simulink model "SWEM_1"  (Simulink 8.6)
settings: Solver=FixedStepAuto  StartTime=0.0  StopTime=100  FixedStep=0.5  MaxStep=dt  RelTol=1e-3
undefined symbols (not defined in the file): fg, kx, ky, Om, phase, phig, PSI_swell, Ua
settings Model: Creator=brynljones  LastModifiedBy=brynljones
settings DataIOCC: SaveFormat=Dataset  SignalLoggingSaveFormat=Dataset
settings OptimizationCC: ExpressionDepthLimit=128
settings DebuggingCC: UnderspecifiedInitializationDetection=Simplified  MergeDetectMultiDrivingBlocksExec=error  SolverPrmCheckMsg=none  FcnCallInpInsideContextMsg=EnableAllAsError  StateNameClashWarn=none
settings HardwareCC: ProdBitPerPointer=64  ProdLargestAtomicFloat=Float  ProdIntDivRoundTo=Zero  ProdEndianess=LittleEndian  ProdWordSize=64  ProdHWDeviceType=Intel->x86-64 (Windows64)
settings GRTTargetCC: GeneratePreprocessorConditionals=Use local settings  CombineOutputUpdateFcns=on  GRTInterface=off
settings ConfigComp: CovModelRefEnable=off

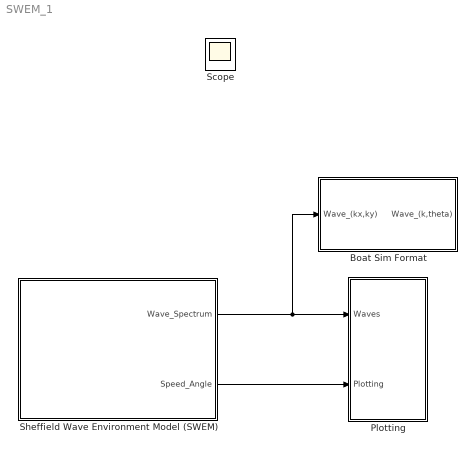
== system SWEM_1 ==
  Boat Sim Format : Subsystem
  Plotting : Subsystem
  Sheffield Wave Environment Model (SWEM) : Subsystem  mask{dt=0.5, M=256, Lx=100*pi, depth=1, lam=5, Viz=Surface Plot, Swell_Hs_u=Swell h_s, Hs_swell=1, U_swell=5, swell_angle=0, fetch_swell=1e10, U_mean=10, wind_angle=30, s=50, GF=1, df=1e-3, Nf=100, mu_wind=1, U_current=0.5, current_angle=-130, mu_current=1}
      mask prompts: dt "Time step (s):"; M "No. gridpoints:"; Lx "Dimension length (m):"; depth "Depth (m):"; lam "Choppy wave factor:"; Viz "Visualisation:"; Swell_Hs_u "Swell windspeed/fetch or h_s:"; Hs_swell "Swell h_s (m):"; U_swell "Swell windspeed (m/s):"; swell_angle "Swell angle (deg):"; fetch_swell "Swell fetch (m):"; U_mean "Mean local windspeed (m/s):"; wind_angle "Mean local wind angle (deg):"; s "Wind wave spreading (s):"; GF "Gust Factor:"; df "Gust freq. spacing:"; Nf "No. of gusting freq. components:"; mu_wind "Wind angle fluctuation coeff:"; U_current "Current speed (m/s):"; current_angle "Mean current angle (deg):"; mu_current "Current angle fluctuation coeff:"
      mask init:
      | if (Swell_Hs_u == 2)
      |     [Om,PSI_swell,kx,ky,phase,U_swell] = swellComponent_Hs(depth,M,M,Lx,Lx,Hs_swell,swell_angle);
      | else
      |     [Om,PSI_swell,kx,ky,phase] = swellComponent_U(depth,M,M,Lx,Lx,U_swell,fetch_swell,swell_angle);
      | end
      | [Ua,phig,fg] = Norso_Gust(U_mean,df,Nf);
      mask TypeOptions Viz: Surface Plot | Contour Plot | No Visualisation
      mask TypeOptions Swell_Hs_u: Swell windspeed/fetch | Swell h_s
      mask Display: image('sea1.jpg')
  Scope : Scope
  wires:
  Sheffield Wave Environment Model (SWEM)/1(Wave_Spectrum) -> Boat Sim Format/1(Wave_(kx,ky)), Plotting/1(Waves)
  Sheffield Wave Environment Model (SWEM)/2(Speed_Angle) -> Plotting/2(Plotting)

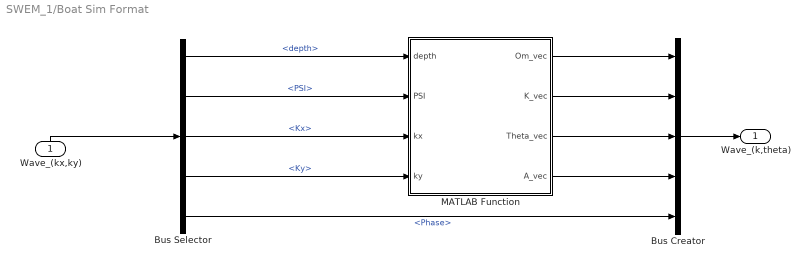
== system SWEM_1/Boat Sim Format ==
  Wave_(kx,ky) : Inport
  Bus Creator : BusCreator  Inputs=5
  Bus Selector : BusSelector  OutputSignals=depth,PSI,Kx,Ky,Phase
  MATLAB Function : MATLAB Function  TreatAsAtomicUnit=on
  Wave_(k,theta) : Outport
  wires:
  Bus Creator/1 -> Wave_(k,theta)/1
  MATLAB Function/2(K_vec) -> Bus Creator/2
  Bus Selector/3 -> MATLAB Function/3(kx)  "<Kx>"
  Bus Selector/4 -> MATLAB Function/4(ky)  "<Ky>"
  Wave_(kx,ky)/1 -> Bus Selector/1
  Bus Selector/2 -> MATLAB Function/2(PSI)  "<PSI>"
  Bus Selector/5 -> Bus Creator/5  "<Phase>"
  MATLAB Function/4(A_vec) -> Bus Creator/4
  MATLAB Function/3(Theta_vec) -> Bus Creator/3
  MATLAB Function/1(Om_vec) -> Bus Creator/1
  Bus Selector/1 -> MATLAB Function/1(depth)  "<depth>"

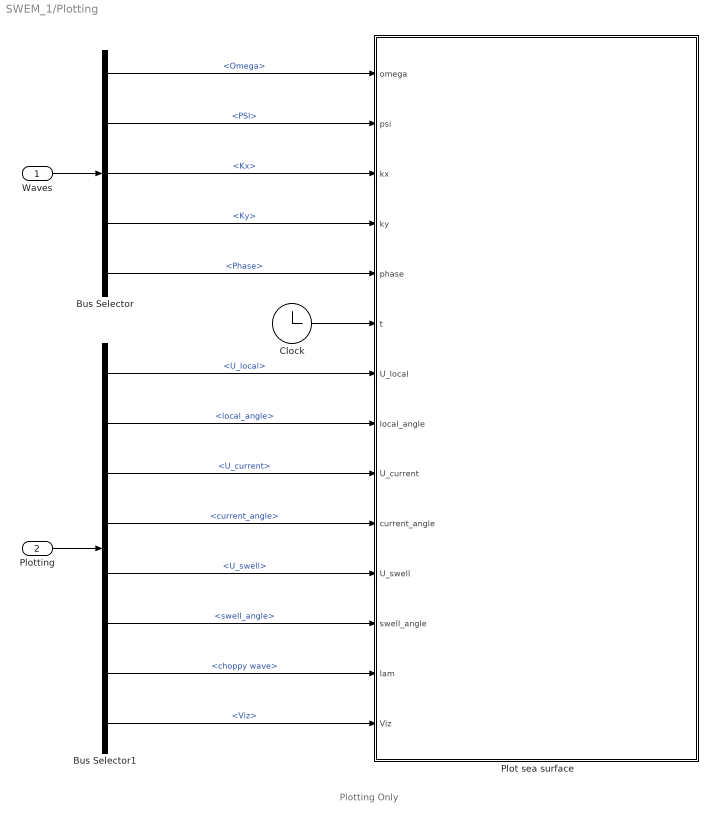
== system SWEM_1/Plotting ==
  note: Plotting Only
  Waves : Inport
  Plotting : Inport  Port=2
  Bus Selector : BusSelector  OutputSignals=Omega,PSI,Kx,Ky,Phase
  Bus Selector1 : BusSelector  OutputSignals=U_local,local_angle,U_current,current_angle,U_swell,swell_angle,choppy wave,Viz
  Clock : Clock
  Plot sea surface : MATLAB Function  TreatAsAtomicUnit=on
  wires:
  Waves/1 -> Bus Selector/1
  Bus Selector1/8 -> Plot sea surface/14(Viz)  "<Viz>"
  Bus Selector/3 -> Plot sea surface/3(kx)  "<Kx>"
  Bus Selector/4 -> Plot sea surface/4(ky)  "<Ky>"
  Bus Selector/5 -> Plot sea surface/5(phase)  "<Phase>"
  Bus Selector/2 -> Plot sea surface/2(psi)  "<PSI>"
  Bus Selector/1 -> Plot sea surface/1(omega)  "<Omega>"
  Plotting/1 -> Bus Selector1/1
  Clock/1 -> Plot sea surface/6(t)
  Bus Selector1/2 -> Plot sea surface/8(local_angle)  "<local_angle>"
  Bus Selector1/1 -> Plot sea surface/7(U_local)  "<U_local>"
  Bus Selector1/4 -> Plot sea surface/10(current_angle)  "<current_angle>"
  Bus Selector1/3 -> Plot sea surface/9(U_current)  "<U_current>"
  Bus Selector1/6 -> Plot sea surface/12(swell_angle)  "<swell_angle>"
  Bus Selector1/5 -> Plot sea surface/11(U_swell)  "<U_swell>"
  Bus Selector1/7 -> Plot sea surface/13(lam)  "<choppy wave>"

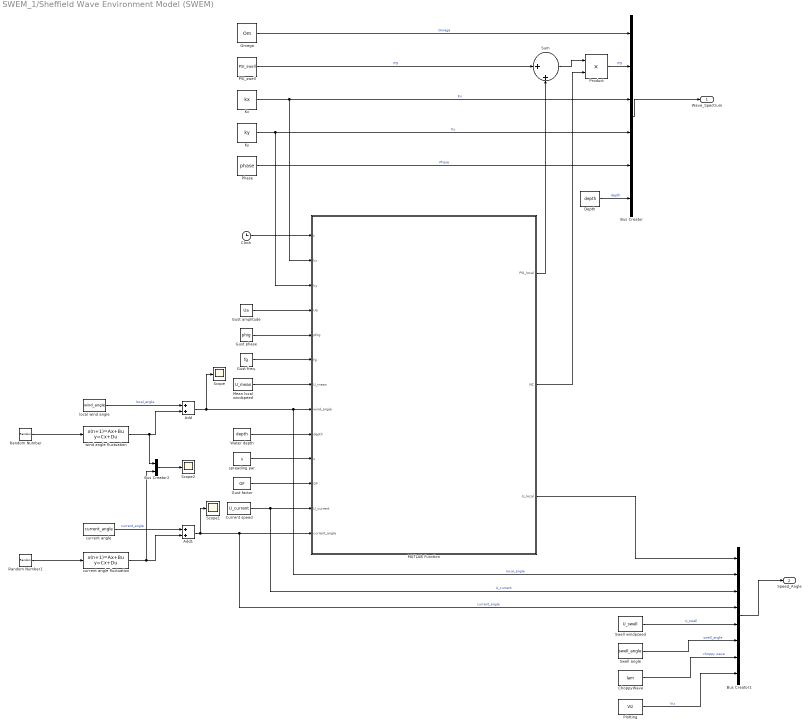
== system SWEM_1/Sheffield Wave Environment Model (SWEM) ==
  Add : Sum
  Add1 : Sum
  Bus Creator : BusCreator  Inputs=6
  Bus Creator1 : BusCreator  Inputs=8
  Bus Creator2 : BusCreator  Inputs=2
  ChoppyWave : Constant  Value=lam
  Clock : Clock
  Current speed : Constant  Value=U_current
  Depth : Constant  Value=depth
  Gust amplitude : Constant  Value=Ua
  Gust factor : Constant  Value=GF
  Gust freq. : Constant  Value=fg
  Gust phase : Constant  Value=phig
  Kx : Constant  Value=kx
  Ky : Constant  Value=ky
  MATLAB Function : MATLAB Function  TreatAsAtomicUnit=on
  Mean local windspeed : Constant  Value=U_mean
  Omega : Constant  Value=Om
  PSI_swell : Constant  Value=PSI_swell
  Phase : Constant  Value=phase
  Plotting : Constant  Value=Viz
  Product : Product
  Random Number : RandomNumber  Variance=5  Seed=2  SampleTime=dt
  Random Number1 : RandomNumber  Variance=2  Seed=1  SampleTime=dt
  Scope : Scope
  Scope1 : Scope
  Scope2 : Scope
  Sum : Sum  Inputs=|++
  Swell angle : Constant  Value=swell_angle
  Swell windpseed : Constant  Value=U_swell
  Water depth : Constant  Value=depth
  current angle : Constant  Value=current_angle
  current angle fluctuation : DiscreteStateSpace  A=1-(dt*mu_current)  B=dt  D=0  X0=-0.3  SampleTime=-1
  local wind angle : Constant  Value=wind_angle
  spreading par. : Constant  Value=s
  wind angle fluctuation : DiscreteStateSpace  A=1-(dt*mu_wind)  B=dt  D=0  X0=0.1  SampleTime=-1
  Wave_Spectrum : Outport
  Speed_Angle : Outport  Port=2
  wires:
  Ky/1 -> MATLAB Function/3(ky), Bus Creator/4  "Ky"
  Phase/1 -> Bus Creator/5  "Phase"
  Omega/1 -> Bus Creator/1  "Omega"
  Kx/1 -> MATLAB Function/2(kx), Bus Creator/3  "Kx"
  Bus Creator/1 -> Wave_Spectrum/1
  Clock/1 -> MATLAB Function/1(t)
  Gust amplitude/1 -> MATLAB Function/4(Ua)
  Gust phase/1 -> MATLAB Function/5(phig)
  Gust freq./1 -> MATLAB Function/6(fg)
  Mean local windspeed/1 -> MATLAB Function/7(U_mean)
  Water depth/1 -> MATLAB Function/9(depth)
  spreading par./1 -> MATLAB Function/10(s)
  Gust factor/1 -> MATLAB Function/11(GF)
  Current speed/1 -> Bus Creator1/3, MATLAB Function/12(U_current)  "U_current"
  MATLAB Function/1(PSI_local) -> Sum/2
  PSI_swell/1 -> Sum/1  "PSI"
  Product/1 -> Bus Creator/2  "PSI"
  MATLAB Function/2(NC) -> Product/2
  Sum/1 -> Product/1
  MATLAB Function/3(U_local) -> Bus Creator1/1
  Swell windpseed/1 -> Bus Creator1/5  "U_swell"
  Swell angle/1 -> Bus Creator1/6  "swell_angle"
  Bus Creator1/1 -> Speed_Angle/1
  Add/1 -> Scope/1, Bus Creator1/2, MATLAB Function/8(wind_angle)  "local_angle"
  local wind angle/1 -> Add/1  "local_angle"
  Random Number/1 -> wind angle fluctuation/1
  wind angle fluctuation/1 -> Bus Creator2/1, Add/2
  Random Number1/1 -> current angle fluctuation/1
  current angle/1 -> Add1/1  "current_angle"
  current angle fluctuation/1 -> Bus Creator2/2, Add1/2
  Add1/1 -> Scope1/1, Bus Creator1/4, MATLAB Function/13(current_angle)  "current_angle"
  Bus Creator2/1 -> Scope2/1
  ChoppyWave/1 -> Bus Creator1/7  "choppy wave"
  Plotting/1 -> Bus Creator1/8  "Viz"
  Depth/1 -> Bus Creator/6  "depth"

== matlab function Sheffield Wave Environment Model (SWEM)/MATLAB Function ==
  data: t input double; PSI_local output double; kx input double; ky input double; Ua input double; phig input double; fg input double; U_mean input double; wind_angle input double; depth input double; s input double; GF input double; U_current input double; current_angle input double; NC output double; U_local output double
function [PSI_local,NC,U_local] = fcn(t,kx,ky,Ua,phig,fg,U_mean,wind_angle,depth,s,GF,U_current,current_angle)
%#codegen


% calculate local wind = mean wind + gust
U_gust = sum(Ua.*cos(2*pi*fg*t + phig*2*pi));
U_local = U_mean + GF*U_gust;
        
% calcuate local wind angle
wind_angle = ((2*pi)/360) * (wind_angle);
 
% calcuate current angle
current_angle = ((2*pi)/360) * (current_angle);

% initialise vectors
PSI_local = zeros(length(kx)*length(ky),1);  % local wind spectrum
NC =zeros(length(kx)*length(ky),1);          % current effects

rw=0;
for mk=1:length(kx)
    for nk=1:length(ky)
        rw=rw+1;       
        
        if (kx(mk)==0 && ky(nk)==0)
            psi_local=0;
            nc = 0;
        else
            [psi_local] = tma_spectrum2(kx(mk),ky(nk),depth,U_local,wind_angle,round(s));
            [nc] = nwogu_current_spec_1(kx(mk),ky(nk),U_current,current_angle,depth);            
        end     
        
        PSI_local(rw) = psi_local;    
        NC(rw) = nc;      
        
    end
end

== matlab function Plotting/Plot sea surface ==
  data: omega input double; psi input double; kx input double; ky input double; phase input double; t input double; U_local input double; local_angle input double; U_current input double; current_angle input double; U_swell input double; swell_angle input double; lam input double; Viz input double
function fcn(omega,psi,kx,ky,phase,t,U_local,local_angle,U_current,current_angle,U_swell,swell_angle,lam,Viz)
%#codegen
coder.extrinsic('sprintf')
coder.extrinsic('compass')
coder.extrinsic('legend')
coder.extrinsic('contourf')
coder.extrinsic('colorbar')
coder.extrinsic('quiver')
coder.extrinsic('annotation')

if (t==0)
    close all
end

if (Viz==3)
    
else
    
    % Parameters
    M = length(kx);
    N = length(ky);
    
    Lx = (2*pi)/kx(2);
    Ly = (2*pi)/ky(2);
    dkx = kx(2);
    dky = ky(2);
    
    x = [0:M-1]*(Lx/M);
    y = [0:N-1]*(Ly/N);
    
    [xx,yy] = meshgrid(x,y);
    [kxx,kyy] = meshgrid(kx,ky);
    kk = sqrt((kxx.^2)+(kyy.^2));
    
    % initialise matrices
    PSI = zeros(M,N);
    Om = zeros(M,N);
    Phase = zeros(M,N);
    
    ind = 0;
    for rw = 1:M
        for col = 1:N
            ind = ind+1;
            
            PSI(rw,col) = psi(ind);
            Om(rw,col) = omega(ind);
            Phase(rw,col) = phase(ind);
            
        end
    end
    
    % calculate aplitude spectrum
    a = sqrt(2*PSI*dkx*dky);
    
    % calculate sig. wave height and sea state
    m0 = sum(sum( (a.^2)/2));
    Hs = 4*sqrt(m0);
    SS = getSS(Hs);
    
    % add time-despendency to ampltide spectrum
    A = a.*exp(1i*(-Om*t + Phase));
    
    KXX = (kxx.*A)./kk;
    KYY = (kyy.*A)./kk;
    
    % calculate x,y,z coordinates of surface
    h = (M*N)*real(ifft2(A));
    
    if (lam>0)
        Dx = (M*N)*imag(ifft2(KXX));
        Dy = (M*N)*imag(ifft2(KYY));
        
        xxn = xx-lam*Dx;
        yyn = yy-lam*Dy;
    else
        xxn = xx;
        yyn = yy;
    end
    
    %% Plotting
    
    % Contour plot
    
    if (Viz==2)
        
       Nx = Lx;

        
        contourf(xxn,yyn,h,20,'linestyle','none');
        caxis([-round(Hs) round(Hs)]);
        colorbar
        colormap('winter')
        xlim([0.05*Nx Lx-0.05*Nx]);
        ylim([0.05*Nx Lx-0.05*Nx]);
        hold on;
        
        Arrow = Nx*(18/(100*pi));
        
        % Swell
        Xswell = (59.1/100)*Nx;
        Yswell = (86/100)*Nx;

        plot([Xswell Xswell],[Yswell Yswell],'ko','markersize',70,'markerfacecolor','white');
        drawArrow([Xswell Xswell+(Arrow*cos(-((2*pi)/360)*swell_angle+pi/2))],[Yswell Yswell+(Arrow*sin(-((2*pi)/360)*swell_angle+pi/2))],'linewidth',1,'color','k','maxheadsize',0.8)
        
        Xswell2 = (55/100)*Nx;
        Yswell2 = (74/100)*Nx;        
        
        Swell_num = sprintf('%3.1f$m/s$',U_swell);        
        text(Xswell2,Yswell2,Swell_num,'interpreter','latex','FontWeight','bold','color','white','fontsize',14);
        
        % Local
        Xlocal = (72.8/100)*Nx;
        Ylocal = (86/100)*Nx;
        
        plot([Xlocal Xlocal],[Ylocal Ylocal],'ko','markersize',70,'markerfacecolor','white');
        drawArrow([Xlocal Xlocal+(Arrow*cos(-((2*pi)/360)*local_angle+pi/2))],[Ylocal Ylocal+(Arrow*sin(-((2*pi)/360)*local_angle+pi/2))],'linewidth',1,'color','k','maxheadsize',0.8)
        
        Xlocal2 = (68.5/100)*Nx;
        Ylocal2 = (74/100)*Nx;
        
        Local_num = sprintf('%3.1f$m/s$',U_local);        
        text(Xlocal2,Ylocal2,Local_num,'interpreter','latex','FontWeight','bold','color','white','fontsize',14);
        
        % Current
        Xc = (86.6/100)*Nx;
        Yc = (86/100)*Nx;
        
        plot([Xc Xc],[Yc Yc],'ko','markersize',70,'markerfacecolor','white');
        drawArrow([Xc Xc+(Arrow*cos(-((2*pi)/360)*current_angle+pi/2))],[Yc Yc+(Arrow*sin(-((2*pi)/360)*current_angle+pi/2))],'linewidth',1,'color','k','maxheadsize',0.8)
        
        Xc2 = (82.5/100)*Nx;
        Yc2 = (74/100)*Nx;       
        
        Current_num = sprintf('%3.1f$m/s$',U_current);        
        text(Xc2,Yc2,Current_num,'interpreter','latex','FontWeight','bold','color','white','fontsize',14);
        
        
        
        
        set(gca,'fontsize',14);
        ylabel('$x$($m$)','interpreter','latex','fontsize',24);
        xlabel('$y$($m$)','interpreter','latex','fontsize',24);
        
        tit = sprintf('$t$=%3.1f$s$, ${h_s}$=%3.2f$m$, Sea State=%i',t,Hs,SS);
        title(tit,'fontsize',20,'interpreter','latex');
        hold off;
        
        
        if (t==0)
            annotation('textbox',[0.52 0.48 0.3 0.3],'String',  'Swell','FontWeight','bold','FitBoxToText','on','edgecolor','none','color','w','backgroundcolor','none');
            annotation('textbox',[0.61 0.48 0.3 0.3],'String','Local wind','FontWeight','bold','FitBoxToText','on','edgecolor','none','color','w','backgroundcolor','none');
            annotation('textbox',[0.73 0.48 0.3 0.3],'String','Current','FontWeight','bold','FitBoxToText','on','edgecolor','none','color','w','backgroundcolor','none');
            
            % Swell
            annotation('textbox',[0.54 0.612 0.3 0.3],'String','0','FitBoxToText','on','edgecolor','none','fontsize',8);
            annotation('textbox',[0.532 0.51 0.3 0.3],'String','180','FitBoxToText','on','edgecolor','none','fontsize',8);
            annotation('textbox',[0.575 0.56 0.3 0.3],'String','90','FitBoxToText','on','edgecolor','none','fontsize',8);
            annotation('textbox',[0.497 0.56 0.3 0.3],'String','270','FitBoxToText','on','edgecolor','none','fontsize',8);
            % Local
            annotation('textbox',[0.65 0.612 0.3 0.3],'String','0','FitBoxToText','on','edgecolor','none','fontsize',8);
            annotation('textbox',[0.642 0.51 0.3 0.3],'String','180','FitBoxToText','on','edgecolor','none','fontsize',8);
            annotation('textbox',[0.685 0.56 0.3 0.3],'String','90','FitBoxToText','on','edgecolor','none','fontsize',8);
            annotation('textbox',[0.607 0.56 0.3 0.3],'String','270','FitBoxToText','on','edgecolor','none','fontsize',8);
            % Current
            annotation('textbox',[0.76 0.612 0.3 0.3],'String','0','FitBoxToText','on','edgecolor','none','fontsize',8);
            annotation('textbox',[0.752 0.51 0.3 0.3],'String','180','FitBoxToText','on','edgecolor','none','fontsize',8);
            annotation('textbox',[0.795 0.56 0.3 0.3],'String','90','FitBoxToText','on','edgecolor','none','fontsize',8);
            annotation('textbox',[0.717 0.56 0.3 0.3],'String','270','FitBoxToText','on','edgecolor','none','fontsize',8);
        end
        
        set(gcf,'position',[100 100 900 700])
        
        drawnow
        
    else
        
        
        
        
        % Surface plot
        subplot(1,2,1)       
        surf(xxn,yyn,h,'linestyle','none');
        
        colormap('winter')
        
        xlim([0 Lx]);
        ylim([0 Ly]);
        zlim([-5*round(Hs) 5*round(Hs)])
        
        caxis([-round(Hs) round(Hs)]);
        
        view([-14 52])
        
        tit = sprintf('$t$=%3.1f$s$, ${h_s}$=%3.2f$m$, Sea State=%i',t,Hs,SS);
        title(tit,'fontsize',20,'interpreter','latex');
        ylabel('$x$($m$)','interpreter','latex','fontsize',24);
        xlabel('$y$($m$)','interpreter','latex','fontsize',24);
        zlabel('$\eta$($m$)','interpreter','latex','fontsize',24);
        set(gca,'fontsize',14);
        
        
        % compass
        subplot(1,2,2)
        if (U_local>U_swell)
            compass(U_local*cos(((2*pi)/360)*local_angle),U_local*sin(((2*pi)/360)*local_angle),'r');
            hold on;
            compass(U_swell*cos(((2*pi)/360)*swell_angle),U_swell*sin(((2*pi)/360)*swell_angle),'b');
            compass(10*U_current*cos(((2*pi)/360)*current_angle),10*U_current*sin(((2*pi)/360)*current_angle),'k');
            hold off;
            legend('Local wind','Swell wind','10xCurrent','Location','south');
            view([90 -90])
        else
            compass(U_swell*cos(((2*pi)/360)*swell_angle),U_swell*sin(((2*pi)/360)*swell_angle),'b');
            hold on;
            compass(U_local*cos(((2*pi)/360)*local_angle),U_local*sin(((2*pi)/360)*local_angle),'r');
            compass(10*U_current*cos(((2*pi)/360)*current_angle),10*U_current*sin(((2*pi)/360)*current_angle),'k');
            hold off;
            legend('Swell wind','Local wind','10xCurrent','Location','south');
            view([90 -90])
        end
        
        drawnow
        
    end
    
end

== matlab function Boat Sim Format/MATLAB Function ==
  data: Om_vec output double; depth input double; PSI input double; K_vec output double; kx input double; ky input double; Theta_vec output double; A_vec output double
% Function converts Wave spectrum from kx,ky to k,theta coordinates

function  [Om_vec,K_vec,Theta_vec,A_vec]= fcn(depth,PSI,kx,ky)
%#codegen

g = 9.81;

% Change matrices so that they are monotonically increasing
[kxx,kyy] = meshgrid(kx,ky);

N = length(kx);
PSI_Mat = zeros(N);

ind = 0;
for rw = 1:N
    for col = 1:N
        ind = ind+1;        
        PSI_Mat(rw,col) = PSI(ind);        
    end
end

kxx2 = [kxx(:,end-(N/2)+2:end) kxx(:,1:(N/2)+1)];
kyy2 = [kyy(:,end-(N/2)+2:end) kyy(:,1:(N/2)+1)];
PSI_2 = [PSI_Mat(:,end-(N/2)+2:end) PSI_Mat(:,1:(N/2)+1)];

kxx3 = [kxx2(end-(N/2)+2:end,:) ; kxx2(1:(N/2)+1,:)];
kyy3 = [kyy2(end-(N/2)+2:end,:) ; kyy2(1:(N/2)+1,:)];
PSI_3 = [PSI_2(end-(N/2)+2:end,:) ; PSI_2(1:(N/2)+1,:)];


% Create k,theta coordinates to interpolate to
kmax = max(kx);
Nk = length(kx);
dk = kmax/Nk;

dthet = (2*pi)/Nk;

k = zeros(Nk,1);
theta = zeros(Nk,1);

for ind=1:Nk
    k(ind) = ind*dk;
    theta(ind) = -pi + (ind*dthet);
end


[Theta,K]=meshgrid(theta,k);
[xp,yp] = pol2cart(Theta,K);

% Interpolate from cartesian to polar
PSI_p = interp2(kxx3,kyy3,PSI_3,xp,yp);


% Save vectors to output
K_vec = zeros(Nk^2,1);
Theta_vec = zeros(Nk^2,1);
PSI_vec = zeros(Nk^2,1);

rw = 0;
for the_i = 1:Nk
    for k_i = 1:Nk
       
        rw = rw+1;
        
        K_vec(rw) = K(the_i,k_i);
        Theta_vec(rw) = Theta(the_i,k_i);
        PSI_vec(rw) = PSI_p(the_i,k_i);
        
    end
end

% Calculate wave amplitudes
A_vec = sqrt(2*PSI_vec.*K_vec*dk*dthet);
Om_vec = sqrt(g*K_vec.*tanh(K_vec*depth));
